simulink model "fullmodel"  (R2021a)
settings: Solver=VariableStepAuto  StartTime=0.0  StopTime=10.0  RelTol=1e-3
undefined symbols (not defined in the file): Fc, Fm, M
libraries: dsparch4 x1
settings Model: Creator=prakh  LastModifiedBy=prakh

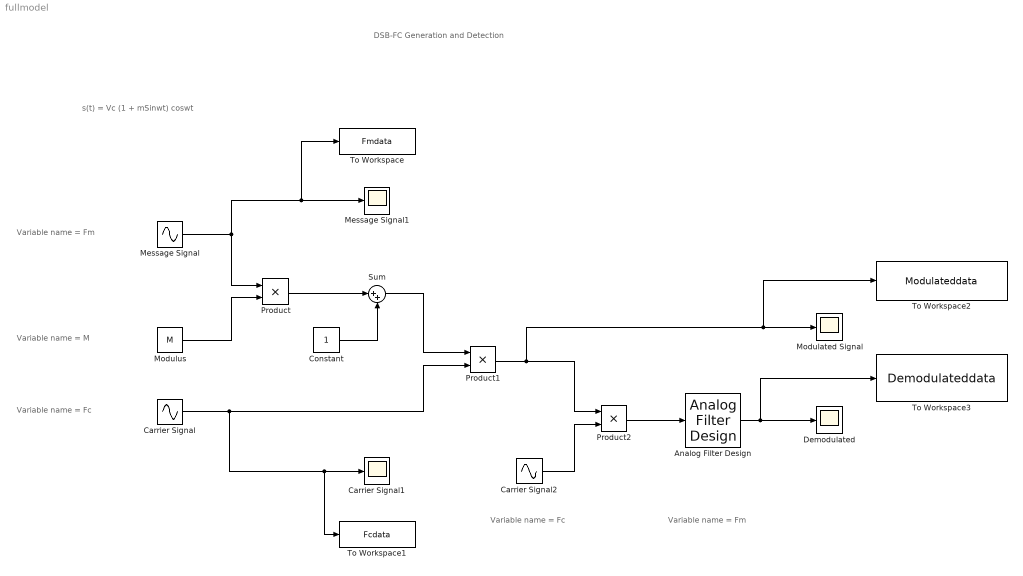
== system fullmodel ==
  note: Variable name = Fm
  note: DSB-FC Generation and Detection
  note: s(t) = Vc (1 + mSinwt) coswt
  note: Variable name = M
  note: Variable name = Fc
  note: Variable name = Fc
  note: Variable name = Fm
  Analog Filter Design : dsparch4/Analog Filter Design  method=Butterworth  filttype=Lowpass  N=8  Wlo=2*pi*Fm  Whi=80  Rp=2  Rs=40
  Carrier Signal : Sin  Frequency=2*pi*Fc  SampleTime=1/1500
  Carrier Signal1 : Scope
  Carrier Signal2 : Sin  Frequency=2*pi*Fc  SampleTime=1/1500
  Constant : Constant
  "Demodulated " : Scope
  Message Signal : Sin  Frequency=2*pi*Fm  SampleTime=1/1500
  Message Signal1 : Scope
  Modulated Signal : Scope
  Modulus : Constant  Value=M
  Product : Product
  Product1 : Product
  Product2 : Product
  Sum : Sum  Inputs=|++
  To Workspace : ToWorkspace  VariableName=Fmdata  SaveFormat=Timeseries  SampleTime=-1
  To Workspace1 : ToWorkspace  VariableName=Fcdata  SaveFormat=Timeseries  SampleTime=-1
  To Workspace2 : ToWorkspace  VariableName=Modulateddata  SaveFormat=Timeseries  SampleTime=-1
  To Workspace3 : ToWorkspace  VariableName=Demodulateddata  SaveFormat=Timeseries  SampleTime=-1
  wires:
  Carrier Signal2/1 -> Product2/2
  Analog Filter Design/1 -> To Workspace3/1, "Demodulated "/1
  Product2/1 -> Analog Filter Design/1
  Sum/1 -> Product1/1
  Product1/1 -> Product2/1, To Workspace2/1, Modulated Signal/1
  Product/1 -> Sum/1
  Carrier Signal/1 -> Product1/2, To Workspace1/1, Carrier Signal1/1
  Constant/1 -> Sum/2
  Modulus/1 -> Product/2
  Message Signal/1 -> To Workspace/1, Message Signal1/1, Product/1
